simulink model "TP_Ericc3_Modele_Matlab_corrige_LMM"  (R2016b)
settings: Solver=VariableStepAuto  StartTime=0.0  StopTime=2.5  FixedStep=0.01  RelTol=1e-4  EnableMultiTasking=on
values from neighbouring files (symbols this model uses):
  Cr = 0.01    [data_modele_eleve.m]
  fv = 1.17*1e-4    (= 0.000117)    [data_modele_eleve.m]
  Jeq = 2.09*1e-5    (= 2.09e-05)    [data_modele_eleve.m]
  KAN = 2*1e6/1080    (= 1851.85185185)    [data_modele_eleve.m]
  Kc =     [data_modele_eleve.m]
  Ki = 0    [data_modele_eleve.m]
  Km = 0.043    [data_modele_eleve.m]
  Kp = 1e6    (= 1000000)    [data_modele_eleve.m]
  Kr =     [data_modele_eleve.m]
  Ks =     [data_modele_eleve.m]
  Kv = 0.17    [data_modele_eleve.m]
settings Model: Creator=Mathieu  LastModifiedBy=emiliendurif
settings DataIOCC: LimitDataPoints=on  SaveFormat=Array
settings OptimizationCC: LifeSpan=inf
settings DebuggingCC: SFUnexpectedBacktrackingDiag=warning  SFNoUnconditionalDefaultTransitionDiag=warning  SFExecutionAtInitializationDiag=none
settings HardwareCC: ProdBitPerPointer=32  ProdBitPerSizeT=32  ProdBitPerPtrDiffT=32  ProdLargestAtomicFloat=None  ProdIntDivRoundTo=Undefined  ProdEndianess=Unspecified  ProdWordSize=32  ProdHWDeviceType=32-bit Generic
settings ModelReferenceCC: PropagateSignalLabelsOutOfModel=off
settings GRTTargetCC: TargetLangStandard=C89/C90 (ANSI)  GeneratePreprocessorConditionals=Disable all
settings ConfigComp: CovMetricSettings=dw  CovHtmlReporting=on  CovSaveCumulativeToWorkspaceVar=on  CovSaveSingleToWorkspaceVar=on  CovExternalEMLEnable=off

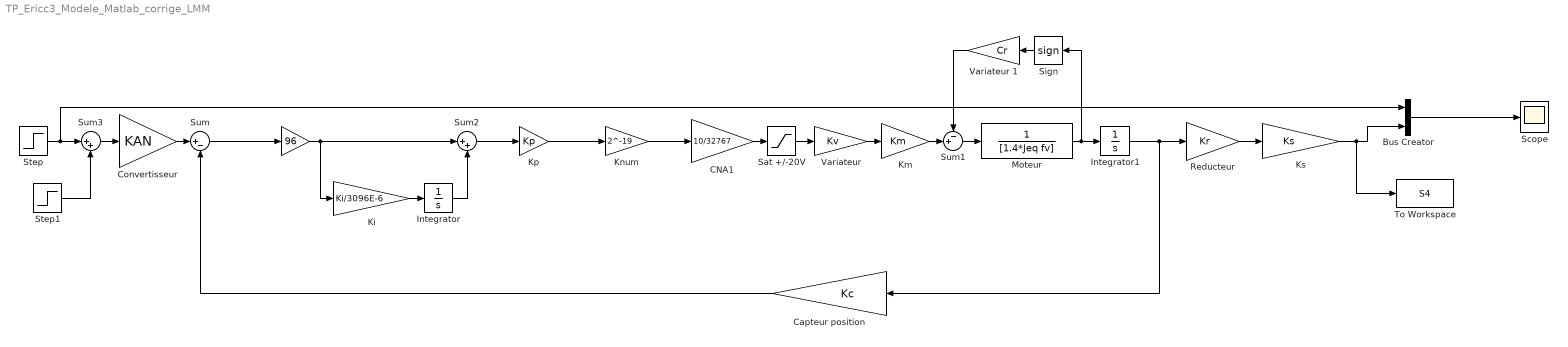
== system TP_Ericc3_Modele_Matlab_corrige_LMM ==
  " " : Gain  Gain=96
  Bus Creator : BusCreator  Inputs=2
  CNA1 : Gain  Gain=10/32767
  "Capteur position " : Gain  Gain=Kc
  Convertisseur : Gain  Gain=KAN
  Integrator : Integrator
  Integrator1 : Integrator
  Ki : Gain  Gain=Ki/3096E-6
  Km : Gain  Gain=Km
  Knum : Gain  Gain=2^-19
  Kp : Gain  Gain=Kp
  Ks : Gain  Gain=Ks
  Moteur : TransferFcn  Denominator=[1.4*Jeq fv]
  Reducteur : Gain  Gain=Kr
  Sat +/-20V : Saturate  UpperLimit=10  LowerLimit=-10
  Scope : Scope
  Sign : Signum
  Step : Step  Time=0  After=30  SampleTime=0  ZeroCross=off
  Step1 : Step  Time=1.1  After=-30  SampleTime=0  ZeroCross=off
  Sum : Sum  Inputs=|+-
  Sum1 : Sum  Inputs=-+|
  Sum2 : Sum  Inputs=|++
  Sum3 : Sum  Inputs=|++
  To Workspace : ToWorkspace  VariableName=S4  SaveFormat=Timeseries  SampleTime=-1
  "Variateur " : Gain  Gain=Kv
  Variateur 1 : Gain  Gain=Cr
  wires:
  Convertisseur/1 -> Sum/1
  Step/1 -> Sum3/1, Bus Creator/1
  "Variateur "/1 -> Km/1
  Km/1 -> Sum1/2
  Moteur/1 -> Sign/1, Integrator1/1
  Integrator1/1 -> "Capteur position "/1, Reducteur/1
  Reducteur/1 -> Ks/1
  Ks/1 -> To Workspace/1, Bus Creator/2
  Bus Creator/1 -> Scope/1
  Sum/1 -> " "/1
  " "/1 -> Ki/1, Sum2/1
  Sum2/1 -> Kp/1
  Integrator/1 -> Sum2/2
  Ki/1 -> Integrator/1
  Sum1/1 -> Moteur/1
  Knum/1 -> CNA1/1
  CNA1/1 -> Sat +/-20V/1
  Sat +/-20V/1 -> "Variateur "/1
  "Capteur position "/1 -> Sum/2
  Kp/1 -> Knum/1
  Sum3/1 -> Convertisseur/1
  Step1/1 -> Sum3/2
  Sign/1 -> Variateur 1/1
  Variateur 1/1 -> Sum1/1
